simulink model "main"  (R2022a)
settings: Solver=ode4  StartTime=0.0  StopTime=10000  FixedStep=0.1  RelTol=1e-3
undefined symbols (not defined in the file or in its folder): X, Y, Z
libraries: nesl_utility x49, sm_lib x23, sharedtransform x3
(part 2 of 2)

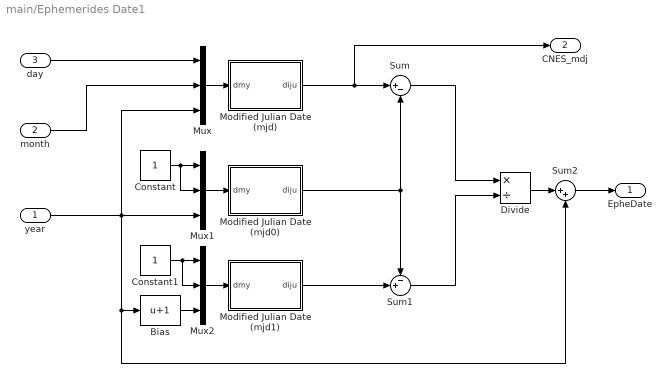
== system main/Ephemerides Date1 ==
  year : Inport
  month : Inport  Port=2
  day : Inport  Port=3
  Bias : Bias  Bias=1  SaturateOnIntegerOverflow=off
  Constant : Constant
  Constant1 : Constant
  Divide : Product  Inputs=*/
  Modified Julian Date (mjd) : MATLAB Function  TreatAsAtomicUnit=on
  Modified Julian Date (mjd0) : MATLAB Function  TreatAsAtomicUnit=on
  Modified Julian Date (mjd1) : MATLAB Function  TreatAsAtomicUnit=on
  Mux : Mux  Inputs=3
  Mux1 : Mux  Inputs=3
  Mux2 : Mux  Inputs=3
  Sum : Sum  Inputs=|+-
  Sum1 : Sum  Inputs=-+|
  Sum2 : Sum  Inputs=|++
  EpheDate : Outport
  CNES_mdj : Outport  Port=2
  wires:
  Sum1/1 -> Divide/2
  Modified Julian Date (mjd1)/1(diju) -> Sum1/2
  month/1 -> Mux/2
  year/1 -> Mux1/3, Mux/3, Bias/1, Sum2/2
  Mux1/1 -> Modified Julian Date (mjd0)/1(dmy)
  day/1 -> Mux/1
  Mux/1 -> Modified Julian Date (mjd)/1(dmy)
  Mux2/1 -> Modified Julian Date (mjd1)/1(dmy)
  Bias/1 -> Mux2/3
  Modified Julian Date (mjd)/1(diju) -> CNES_mdj/1, Sum/1
  Constant1/1 -> Mux2/2, Mux2/1
  Sum/1 -> Divide/1
  Constant/1 -> Mux1/2, Mux1/1
  Modified Julian Date (mjd0)/1(diju) -> Sum1/1, Sum/2
  Divide/1 -> Sum2/1
  Sum2/1 -> EpheDate/1

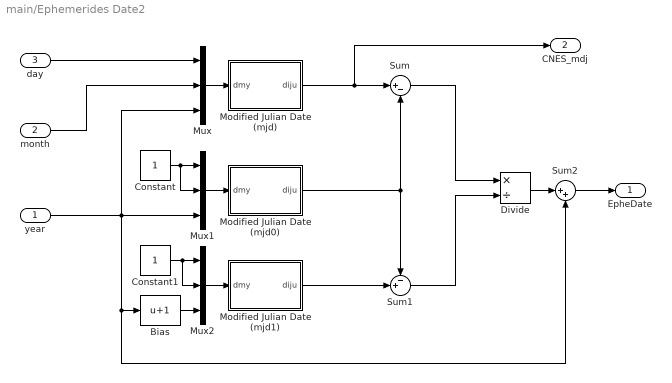
== system main/Ephemerides Date2 ==
  year : Inport
  month : Inport  Port=2
  day : Inport  Port=3
  Bias : Bias  Bias=1  SaturateOnIntegerOverflow=off
  Constant : Constant
  Constant1 : Constant
  Divide : Product  Inputs=*/
  Modified Julian Date (mjd) : MATLAB Function  TreatAsAtomicUnit=on
  Modified Julian Date (mjd0) : MATLAB Function  TreatAsAtomicUnit=on
  Modified Julian Date (mjd1) : MATLAB Function  TreatAsAtomicUnit=on
  Mux : Mux  Inputs=3
  Mux1 : Mux  Inputs=3
  Mux2 : Mux  Inputs=3
  Sum : Sum  Inputs=|+-
  Sum1 : Sum  Inputs=-+|
  Sum2 : Sum  Inputs=|++
  EpheDate : Outport
  CNES_mdj : Outport  Port=2
  wires:
  Sum1/1 -> Divide/2
  Modified Julian Date (mjd1)/1(diju) -> Sum1/2
  month/1 -> Mux/2
  year/1 -> Mux1/3, Mux/3, Bias/1, Sum2/2
  Mux1/1 -> Modified Julian Date (mjd0)/1(dmy)
  day/1 -> Mux/1
  Mux/1 -> Modified Julian Date (mjd)/1(dmy)
  Mux2/1 -> Modified Julian Date (mjd1)/1(dmy)
  Bias/1 -> Mux2/3
  Modified Julian Date (mjd)/1(diju) -> CNES_mdj/1, Sum/1
  Constant1/1 -> Mux2/2, Mux2/1
  Sum/1 -> Divide/1
  Constant/1 -> Mux1/2, Mux1/1
  Modified Julian Date (mjd0)/1(diju) -> Sum1/1, Sum/2
  Divide/1 -> Sum2/1
  Sum2/1 -> EpheDate/1

== matlab function main/Ephemerides Date2/Modified Julian Date (mjd1) ==
  data: dmy input; diju output
function diju  =  djm (dmy)
% [diju] = djm (day, month, year)
%    The function djm furnishes the Modified Julian
%    Date with reference to the day, month and year,
%    at zero hours of the day.
% inputs:
%   dmy(1): day, day of the month
%   dmy(2): month, month of the year
%   dmy(3): year

% outputs:
%   diju
%       Modified Julian Date in days, referred to 1950.0. 
%
% Valdemir Carrara, Apr, 2003
%

diju = 367*dmy(3) + dmy(1) - 712269 + fix(275*dmy(2)/9)- fix(7*(dmy(3)+fix((dmy(2)+9)/12))/4);

== matlab function main/Ephemerides Time2 ==
  data: hours input; dayf output; minutes input; seconds input
function dayf  = time_to_dayf(hours, minutes, seconds)
% [dayf] = time_to_dayf (hours, minutes, seconds)
%    The function time_to_dayf returns with the day elapesed
%    time in seconds
% inputs:
%   hours     
%       day hour (integer).
%   minutes
%       minutes (integer).
%   seconds
%       seconds and fraction of second
% outputs:
%   dayf
%       Day elapsed time in seconds. 
%
% Valdemir Carrara, Feb, 2009
%

dayf = seconds + 60*(minutes + 60*hours);

== matlab function main/Greenwich Aparent Mean Sideral Time1 ==
  data: diju input; gwst output; time input
function gwst  = gst (diju, time)
% [gwst] = gst (diju, time)
%   The function gst furnishes the greenwich aparent mean 
%   sidereal time referred to the J2000.0 equator and equinox.
% inputs:
%   diju
%       Modified Julian Date in days, referred to 1950.0.
%   time
%       UT1 time complement in seconds.
% outputs:
%   gwst
%       Greenwich aparent sidereal time in radians
%
% Valdemir Carrara, Apr, 2003
%

tsj = (diju-18262.5)/36525;
tsgo = (24110.54841 + (8640184.812866 + 9.3104e-2*tsj - 6.2e-6*tsj*tsj)*tsj)*pi/43200;
tetp = 7.292116e-5;		% velocidade angular da Terra (rd/s) mean angular velocity of the Earth
gwst = mod(tsgo + time*tetp, 2*pi);
% reference site
% https://www2.mps.mpg.de/homes/fraenz/systems/systems2art/node10.html
%      if (gwst<0) gwst = gwst + 2*pi

== matlab function main/MATLAB Function6 ==
  data: kepel input; statvec output
function statvec  = kepel_statvec (kepel)
%  [statvec] = kepel_statvec (kepel)
%	The function kepel_statvec transforms the keplerian
%	elements kepel into the corresponding state vector in
%	the same reference system.
%
% Input:
%	kepel
% 		vector containing the keplerian elements:
%		(1) - semimajor axis of the orbit in meters.
%		(2) - eccentricity.
%		(3) - inclinatsion in radians.
%		(4) - right ascension of ascending node in radians.
%		(5) - argument of perigee in radians.
%		(6) - mean anomaly in radians.
% Output:
%	statvec
%  		state vector in meters and meters/second.
%
% Authors:
%	Helio K. Kuga;
%	Valder M. Medeiros;
%	Valdemir Carrara		february/80		version 1.0
%	Valdemir Carrara		july 2005		(C version)
%   Valdemir Carrara            March/09        Matlab

EARTH_GRAVITY	= 3.9860064e+14;		% Earth's gravitational constant (m**3/s**2)

a    = kepel(1);	% semi-major axis
exc  = kepel(2);	% eccentricity

c1   = sqrt(1. - exc*exc);

%     rotation matrix

orb2iner = rotmaz(-kepel(4))*rotmax(-kepel(3))*rotmaz(-kepel(5));

%     Kepler's equation

E    = kepler(kepel(6), exc);

sE   = sin(E);
cE   = cos(E);
c3   = sqrt(EARTH_GRAVITY/a)/(1. - exc*cE);

%     state vector

statvec = [[a*(cE - exc), a*c1*sE, 0]*orb2iner', [-c3*sE, c1*c3*cE, 0]*orb2iner'];

end

function [rot_mat] = rotmax (angle)
% [rot_mat] = rotmax (angle)
%   To obtain the rotation matrix around the X axis given the
%   rotation angle.
% inputs:
%   angle
%       rotation angle, in radians.
% outputs:
%   rot_mat
%       rotation matrix (3, 3)
%

% Valdemir Carrara, Sep, 1998

coan    =  cos(angle);
sian    =  sin(angle);

rot_mat =  [1, 0, 0; 0, coan, sian; 0, -sian, coan];

end

function [rot_mat] = rotmay (angle)
% [rot_mat] = rotmay (angle)
%   To obtain the rotation matrix around the Y axis given the
%   rotation angle.
% inputs:
%   angle
%       rotation angle, in radians.
% outputs:
%   rot_mat
%       rotation matrix (3, 3)
%

% Valdemir Carrara, Sep, 1998


coan    =  cos(angle);
sian    =  sin(angle);

rot_mat =  [coan, 0, -sian; 0, 1, 0; sian, 0, coan];

end

function [rot_mat] = rotmaz (angle)
% [rot_mat] = rotmaz (angle)
%   To obtain the rotation matrix around the Z axis given the
%   rotation angle.
% inputs:
%   angle
%       rotation angle, in radians.
% outputs:
%   rot_mat
%       rotation matrix (3, 3)
%

% Valdemir Carrara, Sep, 1998

coan    =  cos(angle);
sian    =  sin(angle);

rot_mat =  [coan, sian, 0; -sian, coan, 0; 0, 0, 1];
end

function [eccentric] = kepler (mean_anomaly, eccentricity)
% [eccentric] = kepler (mean_anomaly, eccentricity)
%	The subroutine kepler finds a solution to the
%	kepler's equation.
%
% Input:
%	mean_anomaly
%		mean anomaly in radians.
%	eccentricity
%		eccentricity.
%
% Output:
%	eccentric
%		eccentric anomaly in radians.
%
% Authors:
%	Valder M. de Medeiros		june/81		version 2.0
%	Valdemir Carrara			july 2005	(C version)
%   Valdemir Carrara            March/09        Matlab

exc2    = eccentricity*eccentricity;
am1     = mod (mean_anomaly, 2*pi);
am2     = am1 + am1;
am3     = am1 + am2;
shoot   = am1 + eccentricity*(1. - 0.125*exc2)*sin(am1) + ...
		0.5*exc2*(sin(am2) + 0.75*eccentricity*sin(am3));
shoot   = mod (shoot, 2*pi);

e1      = 1.0;
ic      = 0;

while ((abs(e1) > 1.e-12) && (ic <= 10)) 
	e1    = (shoot - am1 - eccentricity*sin(shoot)) / ...
			(1.0 - eccentricity*cos(shoot));
    shoot = shoot - e1;
    ic    = ic + 1;
end

if (ic >= 10)
    disp ('warning ** subroutine kepler did not converge in 10 iterations');
end

eccentric = shoot;


end

== matlab function main/MATLAB Function7 ==
  data: statv input; kepel output
function kepel  = statvec_kepel (statv)
% [kepel] = statvec_kepel (statv)
%
%	The function statvec_kepel transforms the state vector statv
%	into the corresponding keplerian elements in the
%	same reference system.
%
% Input:
%	statv
%		state vector in meters and meters/second.
%
% Output:
%	statvec_kepel
%		vector containing the keplerian elements:
%		(1) - semimajor axis of the orbit in meters.
%		(2) - eccentricity.
%		(3) - inclination in radians.
%		(4) - right ascension of ascending node in radians.
%		(5) - argument of perigee in radians.
%		(6) - mean anomaly in radians.
%
% Authors:
%	Helio K. Kuga
%    Valder M. Medeiros
%	Valdemir Carrara			february/80			version 1.0
%	Helio K. Kuga     			august/82           version 2.0
%	Ulisses T V Guedes 			december/95	 		version 2.1
%               - fix perigee procedure when orbit plane
%                  equal to equatorial plane
%	Valdemir Carrara 			july/05				(C version)
%   Valdemir Carrara            March/09        Matlab

EARTH_GRAVITY	= 3.9860064e+14;		% Earth's gravitational constant (m**3/s**2)

xp  = [statv(1) statv(2) statv(3)];
xv  = [statv(4) statv(5) statv(6)];
r      = sqrt(xp*xp');
vq     = xv*xv';
ainv   = 2.0/r - vq/EARTH_GRAVITY;

h      = cross(xp, xv);
hm     = sqrt(h*h');
an = [0 0 0];
if (hm < 1.e-10)
    disp (' *** Message from function statvec_kepel: *** ');
    disp (' There are no keplerian elements corresponding to this state vector');
    kepel = [0, 0, 0, 0, 0, 0];
else
    h      = h/hm;
    incl   = acos(h(3));
    raan   = atan2(h(1), -h(2));
    d      = xp*xv' / EARTH_GRAVITY;
    esene  = d * sqrt(EARTH_GRAVITY*ainv);
    ecose  = 1 - r*ainv;
    exc    = sqrt(esene*esene + ecose*ecose);
    E      = atan2(esene, ecose);
    mean   = mod (E - esene, 2*pi);
    if mean < 0
        mean = mean + 2*pi;
    end

    if exc < 1.e-10
        arpe = 0;
    else
        dp     = 1./r - ainv;
        ev     = dp*xp - d*xv;
        abev   = sqrt(ev*ev');
        ev     = ev/abev;
        an(1)  = cos(raan);
        an(2)  = sin(raan);
        an(3)  = 0;
        fi     = ev*cross(h, an)';
        arpe = acos(ev*an');
        if fi < 0
            arpe  =  -arpe + 2*pi;
        end
    end

    kepel = [1./ainv, exc, incl, raan, arpe, mean];
end

end

== matlab function main/Ephemerides Date1/Modified Julian Date (mjd) ==
  data: dmy input; diju output
function diju  =  djm (dmy)
% [diju] = djm (day, month, year)
%    The function djm furnishes the Modified Julian
%    Date with reference to the day, month and year,
%    at zero hours of the day.
% inputs:
%   dmy(1): day, day of the month
%   dmy(2): month, month of the year
%   dmy(3): year

% outputs:
%   diju
%       Modified Julian Date in days, referred to 1950.0. 
%
% Valdemir Carrara, Apr, 2003
%

diju = 367*dmy(3) + dmy(1) - 712269 + fix(275*dmy(2)/9)- fix(7*(dmy(3)+fix((dmy(2)+9)/12))/4);

== matlab function main/MATLAB Function8 ==
  data: kepler input; ra output; rp output; T output; T_hour output; we output
function [ra, rp, T, T_hour, we] = fcn(kepler)

u=3.9865*10^14;

a = kepler(1);
e = kepler(2);
% 

ra = a*(1+e);%장반경
rp = a*(1-e);%단반경

a = (ra+rp)/2;% semi-major axis

% a = (550 + 6371.8)*1000;

T = 2*pi*sqrt((a*a*a)/(u));

T_hour = T/3600;

we = 2*pi/T;
% we = 1.1207*0.001;

end

== matlab function main/Ephemerides Date1/Modified Julian Date (mjd0) ==
  data: dmy input; diju output
function diju  =  djm (dmy)
% [diju] = djm (day, month, year)
%    The function djm furnishes the Modified Julian
%    Date with reference to the day, month and year,
%    at zero hours of the day.
% inputs:
%   dmy(1): day, day of the month
%   dmy(2): month, month of the year
%   dmy(3): year

% outputs:
%   diju
%       Modified Julian Date in days, referred to 1950.0. 
%
% Valdemir Carrara, Apr, 2003
%

diju = 367*dmy(3) + dmy(1) - 712269 + fix(275*dmy(2)/9)- fix(7*(dmy(3)+fix((dmy(2)+9)/12))/4);

== matlab function main/MATLAB Function10 ==
  data: stated input; F output
function F = fcn(stated)

accel = [stated(4), stated(5), stated(6)]';
F = accel;
end

== matlab function main/MATLAB Function ==
  data: statv input; kepel output
function kepel  = statvec_kepel (statv)
% [kepel] = statvec_kepel (statv)
%
%	The function statvec_kepel transforms the state vector statv
%	into the corresponding keplerian elements in the
%	same reference system.
%
% Input:
%	statv
%		state vector in meters and meters/second.
%
% Output:
%	statvec_kepel
%		vector containing the keplerian elements:
%		(1) - semimajor axis of the orbit in meters.
%		(2) - eccentricity.
%		(3) - inclination in radians.
%		(4) - right ascension of ascending node in radians.
%		(5) - argument of perigee in radians.
%		(6) - mean anomaly in radians.
%
% Authors:
%	Helio K. Kuga
%    Valder M. Medeiros
%	Valdemir Carrara			february/80			version 1.0
%	Helio K. Kuga     			august/82           version 2.0
%	Ulisses T V Guedes 			december/95	 		version 2.1
%               - fix perigee procedure when orbit plane
%                  equal to equatorial plane
%	Valdemir Carrara 			july/05				(C version)
%   Valdemir Carrara            March/09        Matlab

EARTH_GRAVITY	= 3.9860064e+14;		% Earth's gravitational constant (m**3/s**2)

xp  = [statv(1) statv(2) statv(3)];
xv  = [statv(4) statv(5) statv(6)];
r      = sqrt(xp*xp');
vq     = xv*xv';
ainv   = 2.0/r - vq/EARTH_GRAVITY;

h      = cross(xp, xv);
hm     = sqrt(h*h');
an = [0 0 0];
if (hm < 1.e-10)
    disp (' *** Message from function statvec_kepel: *** ');
    disp (' There are no keplerian elements corresponding to this state vector');
    kepel = [0, 0, 0, 0, 0, 0];
else
    h      = h/hm;
    incl   = acos(h(3));
    raan   = atan2(h(1), -h(2));
    d      = xp*xv' / EARTH_GRAVITY;
    esene  = d * sqrt(EARTH_GRAVITY*ainv);
    ecose  = 1 - r*ainv;
    exc    = sqrt(esene*esene + ecose*ecose);
    E      = atan2(esene, ecose);
    mean   = mod (E - esene, 2*pi);
    if mean < 0
        mean = mean + 2*pi;
    end

    if exc < 1.e-10
        arpe = 0;
    else
        dp     = 1./r - ainv;
        ev     = dp*xp - d*xv;
        abev   = sqrt(ev*ev');
        ev     = ev/abev;
        an(1)  = cos(raan);
        an(2)  = sin(raan);
        an(3)  = 0;
        fi     = ev*cross(h, an)';
        arpe = acos(ev*an');
        if fi < 0
            arpe  =  -arpe + 2*pi;
        end
    end

    kepel = [1./ainv, exc, incl, raan, arpe, mean];
end

end

== matlab function main/Ephemerides Date1/Modified Julian Date (mjd1) ==
  data: dmy input; diju output
function diju  =  djm (dmy)
% [diju] = djm (day, month, year)
%    The function djm furnishes the Modified Julian
%    Date with reference to the day, month and year,
%    at zero hours of the day.
% inputs:
%   dmy(1): day, day of the month
%   dmy(2): month, month of the year
%   dmy(3): year

% outputs:
%   diju
%       Modified Julian Date in days, referred to 1950.0. 
%
% Valdemir Carrara, Apr, 2003
%

diju = 367*dmy(3) + dmy(1) - 712269 + fix(275*dmy(2)/9)- fix(7*(dmy(3)+fix((dmy(2)+9)/12))/4);

== matlab function main/Ephemerides Time1 ==
  data: hours input; dayf output; minutes input; seconds input
function dayf  = time_to_dayf(hours, minutes, seconds)
% [dayf] = time_to_dayf (hours, minutes, seconds)
%    The function time_to_dayf returns with the day elapesed
%    time in seconds
% inputs:
%   hours     
%       day hour (integer).
%   minutes
%       minutes (integer).
%   seconds
%       seconds and fraction of second
% outputs:
%   dayf
%       Day elapsed time in seconds. 
%
% Valdemir Carrara, Feb, 2009
%

dayf = seconds + 60*(minutes + 60*hours);

== matlab function main/MATLAB Function11 ==
  data: stated input; F output
function F = fcn(stated)

accel = [stated(4), stated(5), stated(6)]';
F = accel;
end

== matlab function main/MATLAB Function12 ==
  data: q input; cntl_out output; w input
function cntl_out = LVLH_Attitude_Control(q, w)

qs = q(1);
qv = [q(2), q(3), q(4)]';
w  = [w(1), w(2), w(3)]';

K1 = diag([0.05 0.05 0.05]);
K2 = diag([0.4 0.4 0.4]);

cntl_out = K1*qv - K2*w;

end

== matlab function main/MATLAB Function13 ==
  data: eci2body input; eci2body_X output; eci2body_Y output; eci2body_Z output; eci2lvlh input; eci2lvlh_X output; eci2lvlh_Y output; eci2lvlh_Z output
function [eci2body_X, eci2body_Y, eci2body_Z, eci2lvlh_X, eci2lvlh_Y, eci2lvlh_Z] = fcn(eci2body, eci2lvlh)

eci2body_X = eci2body(:,1);
eci2body_Y = eci2body(:,2);
eci2body_Z = eci2body(:,3);

eci2lvlh_X = eci2lvlh(:,1);
eci2lvlh_Y = eci2lvlh(:,2);
eci2lvlh_Z = eci2lvlh(:,3);

end

== matlab function main/SS Basic Kepler Propagator ==
  data: initial_condition input; dfdt output; eci2lvlh output
function [dfdt, eci2lvlh]   = eq_propagate(initial_condition)

u  = 3.9865*10^14;
Re = 6378137; % earth radius in m
sat_mass = 100;%[kg]

dfdt = zeros(size(initial_condition));

x  = initial_condition(1); % x
y  = initial_condition(2); % y
z  = initial_condition(3); % z
x1 = initial_condition(4); % vel_x
y1 = initial_condition(5); % vel_y
z1 = initial_condition(6); % vel_z

r=sqrt(x^2+y^2+z^2);

% % %   Keplar Motion Equatnion
% % %  => r_dd + u/(r^3)r_ = 0 => r_dd = -u/(r^3)r_
dfdt(1) = x1;% vel_x
dfdt(2) = y1;% vel_y
dfdt(3) = z1;% vel_z
% dfdt(4) = -u*x/r^3 + sat_accel(1) + f_vec(1)/sat_mass;% accel_x
% dfdt(5) = -u*y/r^3 + sat_accel(2) + f_vec(2)/sat_mass;% accel_y
% dfdt(6) = -u*z/r^3 + sat_accel(3) + f_vec(3)/sat_mass;% accel_z
dfdt(4) = -u*x/r^3;% accel_x
dfdt(5) = -u*y/r^3;% accel_y
dfdt(6) = -u*z/r^3;% accel_z

% % % % % % % % % % % % LVLH Frame % % % % % % % % % % % % % % % % % % % % % % % % % % % % % % % % % % % %
% x as the unit vector directed along the spacecraft position vector:
lvlh_z = -[x;y;z]./r; 
rcv    = cross([x;y;z],[x1;y1;z1]);
% z as the unit vector directed along the spacecraft's orbital angular momentum vector:
lvlh_y = rcv/norm(rcv);
% y as the unit vector that completes a right handed coordinate system:
lvlh_x = cross(lvlh_z, lvlh_y);

eci2lvlh = [lvlh_x, lvlh_y, lvlh_z];

end

== matlab function main/MATLAB Function2 ==
  data: kepel input; statvec output
function statvec  = kepel_statvec (kepel)
%  [statvec] = kepel_statvec (kepel)
%	The function kepel_statvec transforms the keplerian
%	elements kepel into the corresponding state vector in
%	the same reference system.
%
% Input:
%	kepel
% 		vector containing the keplerian elements:
%		(1) - semimajor axis of the orbit in meters.
%		(2) - eccentricity.
%		(3) - inclinatsion in radians.
%		(4) - right ascension of ascending node in radians.
%		(5) - argument of perigee in radians.
%		(6) - mean anomaly in radians.
% Output:
%	statvec
%  		state vector in meters and meters/second.
%
% Authors:
%	Helio K. Kuga;
%	Valder M. Medeiros;
%	Valdemir Carrara		february/80		version 1.0
%	Valdemir Carrara		july 2005		(C version)
%   Valdemir Carrara            March/09        Matlab

EARTH_GRAVITY	= 3.9860064e+14;		% Earth's gravitational constant (m**3/s**2)

a    = kepel(1);	% semi-major axis
exc  = kepel(2);	% eccentricity

c1   = sqrt(1. - exc*exc);

%     rotation matrix

orb2iner = rotmaz(-kepel(4))*rotmax(-kepel(3))*rotmaz(-kepel(5));

%     Kepler's equation

E    = kepler(kepel(6), exc);

sE   = sin(E);
cE   = cos(E);
c3   = sqrt(EARTH_GRAVITY/a)/(1. - exc*cE);

%     state vector

statvec = [[a*(cE - exc), a*c1*sE, 0]*orb2iner', [-c3*sE, c1*c3*cE, 0]*orb2iner'];

end

function [rot_mat] = rotmax (angle)
% [rot_mat] = rotmax (angle)
%   To obtain the rotation matrix around the X axis given the
%   rotation angle.
% inputs:
%   angle
%       rotation angle, in radians.
% outputs:
%   rot_mat
%       rotation matrix (3, 3)
%

% Valdemir Carrara, Sep, 1998

coan    =  cos(angle);
sian    =  sin(angle);

rot_mat =  [1, 0, 0; 0, coan, sian; 0, -sian, coan];

end

function [rot_mat] = rotmay (angle)
% [rot_mat] = rotmay (angle)
%   To obtain the rotation matrix around the Y axis given the
%   rotation angle.
% inputs:
%   angle
%       rotation angle, in radians.
% outputs:
%   rot_mat
%       rotation matrix (3, 3)
%

% Valdemir Carrara, Sep, 1998


coan    =  cos(angle);
sian    =  sin(angle);

rot_mat =  [coan, 0, -sian; 0, 1, 0; sian, 0, coan];

end

function [rot_mat] = rotmaz (angle)
% [rot_mat] = rotmaz (angle)
%   To obtain the rotation matrix around the Z axis given the
%   rotation angle.
% inputs:
%   angle
%       rotation angle, in radians.
% outputs:
%   rot_mat
%       rotation matrix (3, 3)
%

% Valdemir Carrara, Sep, 1998

coan    =  cos(angle);
sian    =  sin(angle);

rot_mat =  [coan, sian, 0; -sian, coan, 0; 0, 0, 1];
end

function [eccentric] = kepler (mean_anomaly, eccentricity)
% [eccentric] = kepler (mean_anomaly, eccentricity)
%	The subroutine kepler finds a solution to the
%	kepler's equation.
%
% Input:
%	mean_anomaly
%		mean anomaly in radians.
%	eccentricity
%		eccentricity.
%
% Output:
%	eccentric
%		eccentric anomaly in radians.
%
% Authors:
%	Valder M. de Medeiros		june/81		version 2.0
%	Valdemir Carrara			july 2005	(C version)
%   Valdemir Carrara            March/09        Matlab

exc2    = eccentricity*eccentricity;
am1     = mod (mean_anomaly, 2*pi);
am2     = am1 + am1;
am3     = am1 + am2;
shoot   = am1 + eccentricity*(1. - 0.125*exc2)*sin(am1) + ...
		0.5*exc2*(sin(am2) + 0.75*eccentricity*sin(am3));
shoot   = mod (shoot, 2*pi);

e1      = 1.0;
ic      = 0;

while ((abs(e1) > 1.e-12) && (ic <= 10)) 
	e1    = (shoot - am1 - eccentricity*sin(shoot)) / ...
			(1.0 - eccentricity*cos(shoot));
    shoot = shoot - e1;
    ic    = ic + 1;
end

if (ic >= 10)
    disp ('warning ** subroutine kepler did not converge in 10 iterations');
end

eccentric = shoot;


end

== matlab function main/MATLAB Function1 ==
  data: kepler input; ra output; rp output; T output; T_hour output; we output
function [ra, rp, T, T_hour, we] = fcn(kepler)

u=3.9865*10^14;

a = kepler(1);
e = kepler(2);
% 

ra = a*(1+e);%장반경
rp = a*(1-e);%단반경

a = (ra+rp)/2;% semi-major axis

% a = (550 + 6371.8)*1000;

T = 2*pi*sqrt((a*a*a)/(u));

T_hour = T/3600;

we = 2*pi/T;
% we = 1.1207*0.001;

end

== matlab function main/MATLAB Function4 ==
  data: eci2body input; eci2body_X output; eci2body_Y output; eci2body_Z output; eci2lvlh input; eci2lvlh_X output; eci2lvlh_Y output; eci2lvlh_Z output
function [eci2body_X, eci2body_Y, eci2body_Z, eci2lvlh_X, eci2lvlh_Y, eci2lvlh_Z] = fcn(eci2body, eci2lvlh)

eci2body_X = eci2body(:,1);
eci2body_Y = eci2body(:,2);
eci2body_Z = eci2body(:,3);

eci2lvlh_X = eci2lvlh(:,1);
eci2lvlh_Y = eci2lvlh(:,2);
eci2lvlh_Z = eci2lvlh(:,3);

end

== matlab function main/MATLAB Function9 ==
  data: ss_state input; ss_stated input; relative_r output; ts_state input; relative_v output; ts_stated input; relative_a output
function [relative_r, relative_v, relative_a] = fcn(ss_state, ss_stated, ts_state, ts_stated)

ss_r = [ss_state(1), ss_state(2), ss_state(3)]';
ss_v = [ss_state(4), ss_state(5), ss_state(6)]';
ss_a = [ss_stated(1), ss_stated(2), ss_stated(3)]';
ts_r = [ts_state(1), ts_state(2), ts_state(3)]';
ts_v = [ts_state(4), ts_state(5), ts_state(6)]';
ts_a = [ts_stated(1), ts_stated(2), ts_stated(3)]';

relative_r = ts_r - ss_r;
relative_v = ts_v - ss_v;
relative_a = ts_a - ss_a;
end

== matlab function main/Greenwich Aparent Mean Sideral Time ==
  data: diju input; gwst output; time input
function gwst  = gst (diju, time)
% [gwst] = gst (diju, time)
%   The function gst furnishes the greenwich aparent mean 
%   sidereal time referred to the J2000.0 equator and equinox.
% inputs:
%   diju
%       Modified Julian Date in days, referred to 1950.0.
%   time
%       UT1 time complement in seconds.
% outputs:
%   gwst
%       Greenwich aparent sidereal time in radians
%
% Valdemir Carrara, Apr, 2003
%

tsj = (diju-18262.5)/36525;
tsgo = (24110.54841 + (8640184.812866 + 9.3104e-2*tsj - 6.2e-6*tsj*tsj)*tsj)*pi/43200;
tetp = 7.292116e-5;		% velocidade angular da Terra (rd/s) mean angular velocity of the Earth
gwst = mod(tsgo + time*tetp, 2*pi);
% reference site
% https://www2.mps.mpg.de/homes/fraenz/systems/systems2art/node10.html
%      if (gwst<0) gwst = gwst + 2*pi

== matlab function main/TS Basic Kepler Propagator ==
  data: initial_condition input; dfdt output; eci2lvlh output
function [dfdt, eci2lvlh]   = eq_propagate(initial_condition)

u  = 3.9865*10^14;
Re = 6378137; % earth radius in m
sat_mass = 100;%[kg]

dfdt = zeros(size(initial_condition));

x  = initial_condition(1); % x
y  = initial_condition(2); % y
z  = initial_condition(3); % z
x1 = initial_condition(4); % vel_x
y1 = initial_condition(5); % vel_y
z1 = initial_condition(6); % vel_z

r=sqrt(x^2+y^2+z^2);

% % %   Keplar Motion Equatnion
% % %  => r_dd + u/(r^3)r_ = 0 => r_dd = -u/(r^3)r_
dfdt(1) = x1;% vel_x
dfdt(2) = y1;% vel_y
dfdt(3) = z1;% vel_z
% dfdt(4) = -u*x/r^3 + sat_accel(1) + f_vec(1)/sat_mass;% accel_x
% dfdt(5) = -u*y/r^3 + sat_accel(2) + f_vec(2)/sat_mass;% accel_y
% dfdt(6) = -u*z/r^3 + sat_accel(3) + f_vec(3)/sat_mass;% accel_z
dfdt(4) = -u*x/r^3;% accel_x
dfdt(5) = -u*y/r^3;% accel_y
dfdt(6) = -u*z/r^3;% accel_z

% % % % % % % % % % % % LVLH Frame % % % % % % % % % % % % % % % % % % % % % % % % % % % % % % % % % % % %
% x as the unit vector directed along the spacecraft position vector:
lvlh_z = -[x;y;z]./r; 
rcv    = cross([x;y;z],[x1;y1;z1]);
% z as the unit vector directed along the spacecraft's orbital angular momentum vector:
lvlh_y = rcv/norm(rcv);
% y as the unit vector that completes a right handed coordinate system:
lvlh_x = cross(lvlh_z, lvlh_y);

eci2lvlh = [lvlh_x, lvlh_y, lvlh_z];

end

== matlab function main/Ephemerides Date2/Modified Julian Date (mjd) ==
  data: dmy input; diju output
function diju  =  djm (dmy)
% [diju] = djm (day, month, year)
%    The function djm furnishes the Modified Julian
%    Date with reference to the day, month and year,
%    at zero hours of the day.
% inputs:
%   dmy(1): day, day of the month
%   dmy(2): month, month of the year
%   dmy(3): year

% outputs:
%   diju
%       Modified Julian Date in days, referred to 1950.0. 
%
% Valdemir Carrara, Apr, 2003
%

diju = 367*dmy(3) + dmy(1) - 712269 + fix(275*dmy(2)/9)- fix(7*(dmy(3)+fix((dmy(2)+9)/12))/4);

== matlab function main/Ephemerides Date2/Modified Julian Date (mjd0) ==
  data: dmy input; diju output
function diju  =  djm (dmy)
% [diju] = djm (day, month, year)
%    The function djm furnishes the Modified Julian
%    Date with reference to the day, month and year,
%    at zero hours of the day.
% inputs:
%   dmy(1): day, day of the month
%   dmy(2): month, month of the year
%   dmy(3): year

% outputs:
%   diju
%       Modified Julian Date in days, referred to 1950.0. 
%
% Valdemir Carrara, Apr, 2003
%

diju = 367*dmy(3) + dmy(1) - 712269 + fix(275*dmy(2)/9)- fix(7*(dmy(3)+fix((dmy(2)+9)/12))/4);
